simulink model "feedback_control"  (R2024a)
settings: Solver=FixedStepDiscrete  StartTime=0.0  StopTime=Inf  FixedStep=T_sample_control  RelTol=1e-3  EnableMultiTasking=on
undefined symbols (not defined in the file): Down, GPTRIP1SEL, T_sample_control, TZ1, Up
libraries: c2802xlib x7, c280xlib x4, c2837xDlib x4, simulink x3, mcbpositiondecoderlib x2, c2000lib x1
settings Model: DataDictionary=pid.sldd  EnableAccessToBaseWorkspace=off  ModifiedByFormat=The MathWorks Inc.  ExtModeTrigDuration=8  Creator=The MathWorks, Inc.  LastModifiedBy=The MathWorks Inc.
settings SolverCC: AlgebraicLoopSolver=TrustRegion  AutoInsertRateTranBlk=on
settings DataIOCC: SaveFormat=Array  ReturnWorkspaceOutputs=off
settings OptimizationCC: DefaultUnderspecifiedDataType=single  EnhancedBackFolding=on  PassReuseOutputArgsAs=Individual arguments  ExpressionDepthLimit=2147483647  EfficientFloat2IntCast=on  LifeSpan=1  MaxStackSize=1024  OptimizeBlockOrder=speed  DifferentSizesBufferReuse=on  OptimizationCustomize=off  EfficientTunableParamExpr=on
settings DebuggingCC: SolverPrmCheckMsg=warning  ParamSuppressDoubleToSinglePrecisionLossMsg=on  FcnCallInpInsideContextMsg=warning  UnconnectedInputMsg=warning  UnconnectedOutputMsg=warning  UnconnectedLineMsg=warning  UniqueDataStoreMsg=error  AssertControl=DisableAll  AllowSymbolicDim=off  StateNameClashWarn=warning  StrictBusMsg=ErrorOnBusTreatedAsVector  SFUnexpectedBacktrackingDiag=warning  SFNoUnconditionalDefaultTransitionDiag=warning  SFExecutionAtInitializationDiag=none  ArithmeticOperatorsInVariantConditions=warning
settings HardwareCC: ProdBitPerChar=16  ProdBitPerInt=16  ProdBitPerPointer=32  ProdBitPerSizeT=32  ProdBitPerPtrDiffT=32  ProdLargestAtomicInteger=Integer  ProdLargestAtomicFloat=None  ProdWordSize=16  ProdLongLongMode=on  ProdHWDeviceType=Texas Instruments->C2000  HardwareBoardFeatureSet=SoCBlockset
settings ModelReferenceCC: EnableRefExpFcnMdlSchedulingChecks=on  PropagateSignalLabelsOutOfModel=off
settings SFSimCC: SimUseLocalCustomCode=off  CustomCodeUndefinedFunction=UseInterfaceOnly
settings RTWCC: Description=Embedded Coder  SystemTargetFile=ert.tlc  HardwareBoard=TI Delfino F28379D LaunchPad  TemplateMakefile=ert_default_tmf  RTWUseLocalCustomCode=off  Toolchain=Texas Instruments Code Composer Studio (C2000)  IncludeHyperlinkInReport=on  CodeProfilingSaveOptions=MetricsOnly  GPUComputeCapability=3.5
settings CodeAppCC: IgnoreCustomStorageClasses=off  CustomSymbolStrType=$N$R$M  StateflowObjectComments=on  InternalIdentifier=Classic
settings ERTTargetCC: CodeReplacementLibrary=TI C28x  MultiwordLength=2048  ParenthesesLevel=Maximum  ExtModeTransport=4  ExtModeStaticAlloc=on  ExtModeAutomaticAllocSize=off  ExtModeStaticAllocSize=10000  ExtModeMexFile=ext_xcp  ExtModeIntrfLevel=Level2 - Open  ConvertIfToSwitch=off  SuppressUnreachableDefaultCases=off
settings ConfigComp: CovMetricSettings=dw  CovSaveCumulativeToWorkspaceVar=on  CovSaveSingleToWorkspaceVar=on  CovExternalEMLEnable=off  CovSFcnEnable=off

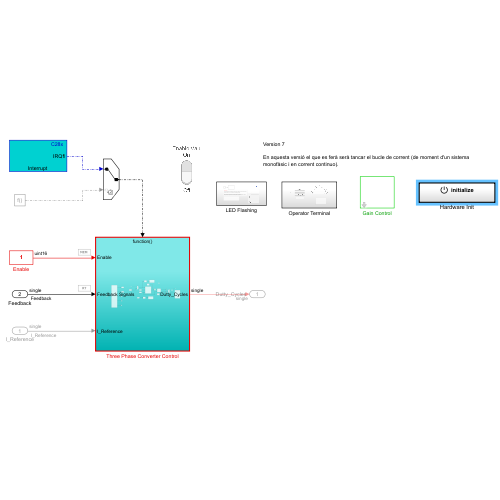
[thumbnail: Simulink's stored preview of the top-level diagram]
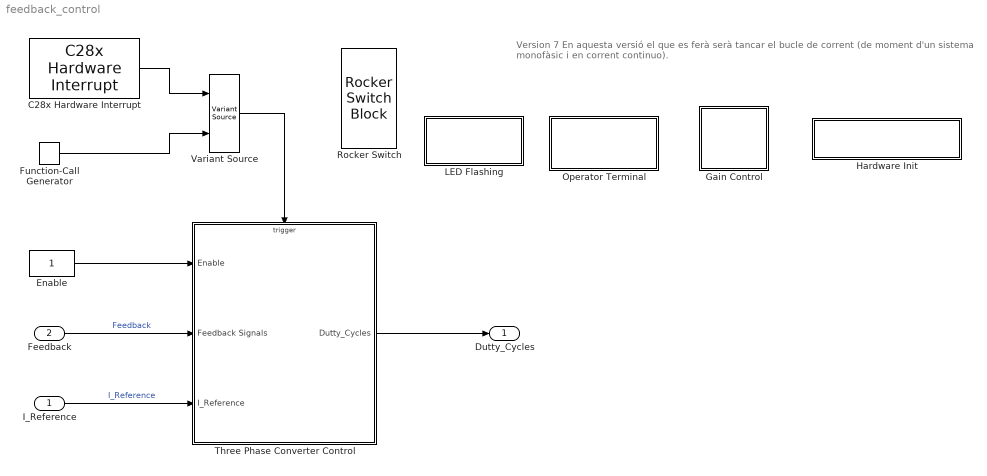
== system feedback_control ==
  note: Version 7
      |
      | En aquesta versió el que es ferà serà tancar el bucle de corrent (de moment d'un sistema monofàsic i en corrent continuo).
  I_Reference : Inport  OutDataTypeStr=single  PortDimensions=1  SampleTime=T_sample_control
  Feedback : Inport  Port=2  OutDataTypeStr=single  PortDimensions=3  SampleTime=T_sample_control
  C28x Hardware Interrupt : c2000lib/Scheduling/C28x Hardware Interrupt  irqnumbers=[1]  pienumbers=[1]  irqpriorities=[30]  irqpreempts=[1]  showinput=off  dspchiptype=C280X
  Enable : Constant  OutDataTypeStr=Inherit: Inherit via back propagation  SampleTime=-1
  Function-Call Generator : simulink/Ports & Subsystems/Function-Call Generator  sample_time=1/10000  numberOfIterations=1  DisallowWideOutput=off
  Gain Control : Subsystem  mask{Gain_Text_R=80 V/V, Gain_Text_S=80 V/V, Gain_Text_T=80 V/V}
      mask prompts: Gain_Text_R "Gain V/V:"; Gain_Text_S "Gain V/V:"; Gain_Text_T "Gain V/V:"
      mask init:
      | Gain_R = Gain_Text_R - 1;
      | Gain_S = Gain_Text_S - 1;
      | Gain_T = Gain_Text_T - 1;
      mask TypeOptions Gain_Text_R: 10 V/V | 20 V/V | 40 V/V | 80 V/V
      mask TypeOptions Gain_Text_S: 10 V/V | 20 V/V | 40 V/V | 80 V/V
      mask TypeOptions Gain_Text_T: 10 V/V | 20 V/V | 40 V/V | 80 V/V
  Hardware Init : Subsystem  TreatAsAtomicUnit=on
  LED Flashing : Subsystem
  Operator Terminal : Subsystem
  Rocker Switch : RockerSwitchBlock
      settings: Values={{'Off', 'On'}, [0 1]}
  Three Phase Converter Control : Subsystem
  Variant Source : VariantSource  VariantControlMode=sim codegen switching  OutputFunctionCall=on
  Dutty_Cycles : Outport  OutDataTypeStr=single  PortDimensions=3  SampleTime=T_sample_control
  wires:
  I_Reference/1 -> Three Phase Converter Control/3(I_Reference)  "I_Reference"
  Enable/1 -> Three Phase Converter Control/1(Enable)
  Feedback/1 -> Three Phase Converter Control/2(Feedback Signals)  "Feedback"
  Three Phase Converter Control/1(Dutty_Cycles) -> Dutty_Cycles/1
  C28x Hardware Interrupt/1 -> Variant Source/1
  Function-Call Generator/1 -> Variant Source/2
  Variant Source/1 -> Three Phase Converter Control/Trigger

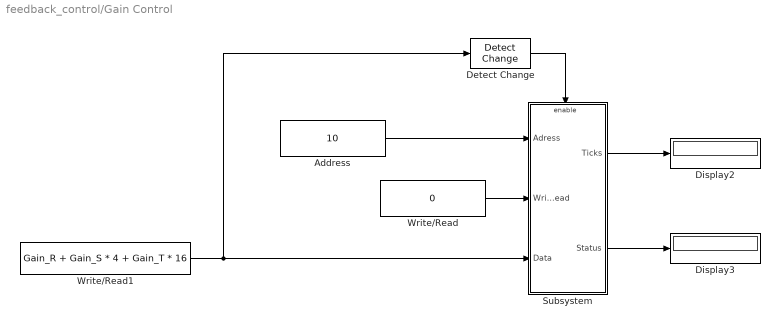
== system feedback_control/Gain Control ==
  Address : Constant  Value=10  OutDataTypeStr=uint16  SampleTime=-1
  Detect Change : simulink/Logic and Bit Operations/Detect Change  vinit=0  OutDataTypeStr=boolean
  Display2 : Display
  Display3 : Display
  Subsystem : Subsystem
  Write/Read : Constant  Value=0  OutDataTypeStr=uint16  SampleTime=-1
  Write/Read1 : Constant  Value=Gain_R + Gain_S * 4 + Gain_T * 16  OutDataTypeStr=uint16  SampleTime=-1
  wires:
  Detect Change/1 -> Subsystem/Enable
  Write/Read1/1 -> Detect Change/1, Subsystem/3(Data)
  Write/Read/1 -> Subsystem/2(Write/Read)
  Subsystem/2(Status) -> Display3/1
  Subsystem/1(Ticks) -> Display2/1
  Address/1 -> Subsystem/1(Adress)

== system feedback_control/Hardware Init ==
  Event Listener : EventListener  DisableCoverage=on  EventName=reset
  HW_Init : Subsystem  Variant=on  VariantControlMode=sim codegen switching

== system feedback_control/LED Flashing ==
  note: In the GPIO DO (Digital Output) instruction, a part from selecting the GPIO31, we will select the Toggle GPIO31, which means that every time we write a 1 to the position of the corresponding GPIO, it will toggle it state.
  note: Flashing LED
      |
      | The Launchpad used in this laboratory, has a blue LED, which we will turn on and off at a frequency of 2 Hz (every 1/2 second, the LED will trogle it state).
      |
      | At the figure at your right, there is the schematic of the Launchpad, where one can see that the LED D10 is connected to the GPIO31 ( General Purpose I/O ).
  Constant : Constant  OutDataTypeStr=single  SampleTime=0.5
  Digital Output1 : c2837xDlib/Digital Output  GPIO_Number=GPIO24~GPIO31  GPIO_Bit0=off  GPIO_BIT0_Toggle=off  GPIO_Bit1=off  GPIO_BIT1_Toggle=off  GPIO_Bit2=off  GPIO_BIT2_Toggle=off  GPIO_Bit3=off  GPIO_BIT3_Toggle=off  GPIO_Bit4=off  GPIO_BIT4_Toggle=off  GPIO_Bit5=off  GPIO_BIT5_Toggle=off  GPIO_Bit6=off  GPIO_BIT6_Toggle=off  GPIO_Bit7=on  GPIO_BIT7_Toggle=on
  wires:
  Constant/1 -> Digital Output1/1

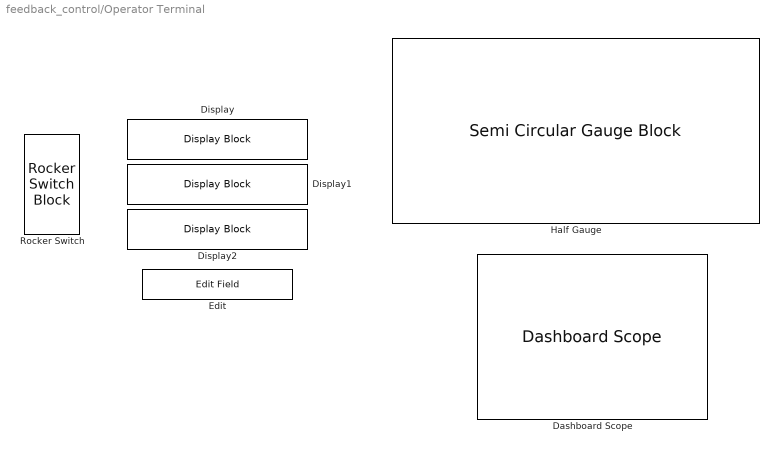
== system feedback_control/Operator Terminal ==
  Dashboard Scope : DashboardScope
  Display : DisplayBlock  Transparency=1
  Display1 : DisplayBlock  Transparency=1
  Display2 : DisplayBlock  Transparency=1
  Edit : EditField  LabelPosition=Hide  ShowInitialText=on  Alignment=Center
  Half Gauge : SemiCircularGaugeBlock  ScaleMax=50
  Rocker Switch : RockerSwitchBlock
      settings: Values={{'Off', 'On'}, [0 1]}

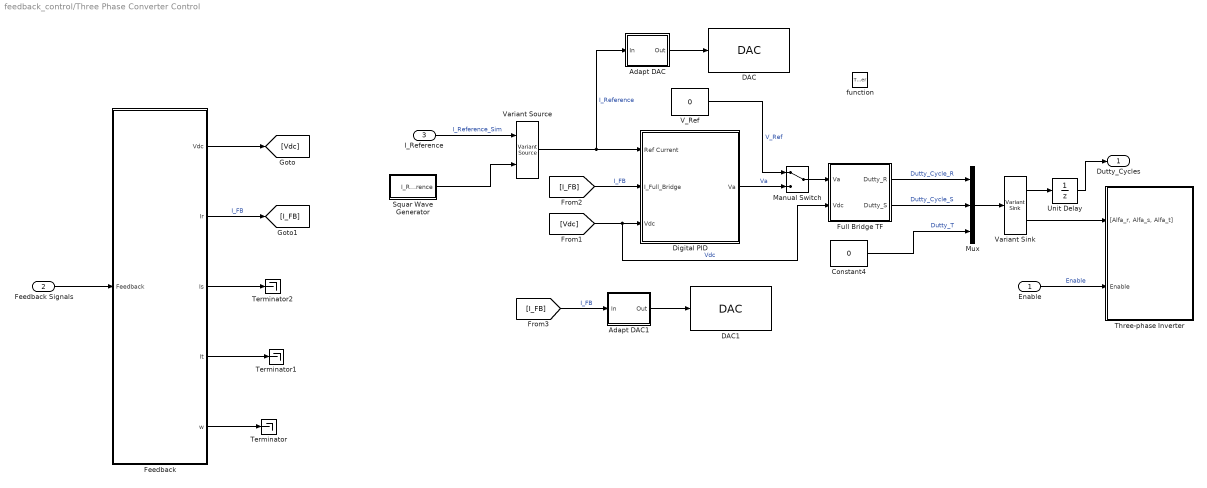
== system feedback_control/Three Phase Converter Control ==
  Enable : Inport
  Feedback Signals : Inport  Port=2
  I_Reference : Inport  Port=3
  function : TriggerPort  TriggerType=function-call  VariantControl=Variant  DisallowConstTsAndPrmTs=on
  Adapt DAC : Subsystem  mask{Offset=(3.3/3)*2048, Gain=(67.0/5.0)*(3/4095.0)}
  Adapt DAC1 : Subsystem  mask{Offset=2048, Gain=(2047*0.007*20*10)/1.65}
  Constant4 : Constant  Value=0  OutDataTypeStr=Inherit: Inherit via back propagation  SampleTime=-1
  DAC : c2837xDlib/DAC  channel=A  saturate=off
  DAC1 : c2837xDlib/DAC  channel=B  saturate=off
  Digital PID : Subsystem  mask{Kp=(2*15-1)*705e-3, Ki=2*15*15*705e-3*705e-3/9.05e-3, max=590, F=10}
      mask prompts: Kp "Proportional:"; Ki "Intragrator constant:"; max "Maximum Voltage:"; F "Sampling Frequency (hKz):"
      mask init:
      | Ts = 1 / (F * 1000);
  Feedback : Subsystem  Variant=on  VariantControlMode=sim codegen switching
  Full Bridge TF : Subsystem
  Manual Switch : ManualSwitch
  Mux : Mux  Inputs=3
  Squar Wave Generator : Subsystem
  Terminator : Terminator
  Terminator1 : Terminator
  Terminator2 : Terminator
  Three-phase Inverter : Subsystem  mask{Fcomm=10, FClk=100}
      mask prompts: Fcomm "Enter the Commutation Frequency (kHz):"; FClk "Enter the Clock Frequency of the CPU (MHz):"
      mask init:
      | Period = (FClk*1000)/(2*Fcomm);
  Unit Delay : UnitDelay  SampleTime=-1  HasFrameUpgradeWarning=on
  V_Ref : Constant  Value=0  OutDataTypeStr=Inherit: Inherit via back propagation  SampleTime=-1
  Variant Sink : VariantSink  VariantControlMode=sim codegen switching
  Variant Source : VariantSource  VariantControlMode=sim codegen switching
  Dutty_Cycles : Outport
  wires:
  [Vdc] -> Digital PID/3(Vdc), Full Bridge TF/2(Vdc)  "Vdc"
  Enable/1 -> Three-phase Inverter/2(Enable)  "Enable"
  Constant4/1 -> Mux/3  "Dutty_T"
  Variant Sink/2 -> Three-phase Inverter/1("[Alfa_r, Alfa_s, Alfa_t]")
  Feedback Signals/1 -> Feedback/1(Feedback)
  Variant Sink/1 -> Unit Delay/1
  Variant Source/1 -> Digital PID/1(Ref Current), Adapt DAC/1(In)  "I_Reference"
  Feedback/2(Ir) -> [I_FB]  "I_FB"
  Feedback/3(Is) -> Terminator2/1
  Feedback/4(It) -> Terminator1/1
  Feedback/5(w) -> Terminator/1
  Mux/1 -> Variant Sink/1
  Full Bridge TF/1(Dutty_R) -> Mux/1  "Dutty_Cycle_R"
  Full Bridge TF/2(Dutty_S) -> Mux/2  "Dutty_Cycle_S"
  Feedback/1(Vdc) -> [Vdc]
  [I_FB] -> Digital PID/2(I_Full_Bridge)  "I_FB"
  Unit Delay/1 -> Dutty_Cycles/1
  I_Reference/1 -> Variant Source/1  "I_Reference_Sim"
  Squar Wave Generator/1(I_Reference) -> Variant Source/2
  Digital PID/1(Va) -> Manual Switch/2  "Va"
  Manual Switch/1 -> Full Bridge TF/1(Va)
  V_Ref/1 -> Manual Switch/1  "V_Ref"
  Adapt DAC/1(Out) -> DAC/1
  Adapt DAC1/1(Out) -> DAC1/1
  [I_FB] -> Adapt DAC1/1(In)  "I_FB"

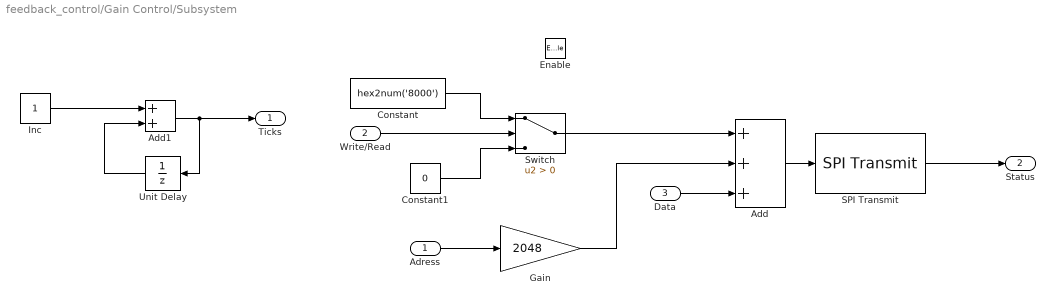
== system feedback_control/Gain Control/Subsystem ==
  Adress : Inport
  Write/Read : Inport  Port=2
  Data : Inport  Port=3
  Enable : EnablePort
  Add : Sum  Inputs=+++  AccumDataTypeStr=uint16
  Add1 : Sum
  Constant : Constant  Value=hex2num('8000')  OutDataTypeStr=uint16  SampleTime=-1
  Constant1 : Constant  Value=0  OutDataTypeStr=uint16  SampleTime=-1
  Gain : Gain  Gain=2048  ParamDataTypeStr=uint16  OutDataTypeStr=uint16
  Inc : Constant  OutDataTypeStr=uint16  SampleTime=-1
  SPI Transmit : c280xlib/SPI Transmit  SPISelect=SPI_A  ClockPolarity=Rising_edge  ClockPhase=No_delay  SPIModule=uint32(0)  Mode=Master  BusSpeed=uint32(1000000)  FirstBitToTransfer=Most significant bit (MSB)  ClockMode=0  BlockFunction=Write  EnableRegisterAddress=on  RegisterAddress=0  OutputDataType=int8  OutputDataLength=1  BlockingMode=off  DataBits=16  UseCustomSSPin=Provided by the SPI peripheral  ActiveLowSSPin=Active low  Pin=0
  Switch : Switch  Criteria=u2 > Threshold  SaturateOnIntegerOverflow=off  InputSameDT=off
  Unit Delay : UnitDelay  SampleTime=-1  StateName=Ticks  HasFrameUpgradeWarning=on
  Ticks : Outport  VectorParamsAs1DForOutWhenUnconnected=off
  Status : Outport  Port=2  VectorParamsAs1DForOutWhenUnconnected=off
  wires:
  Constant1/1 -> Switch/3
  Constant/1 -> Switch/1
  Write/Read/1 -> Switch/2
  Adress/1 -> Gain/1
  Switch/1 -> Add/1
  Gain/1 -> Add/2
  Add/1 -> SPI Transmit/1
  SPI Transmit/1 -> Status/1
  Add1/1 -> Ticks/1, Unit Delay/1
  Unit Delay/1 -> Add1/2
  Inc/1 -> Add1/1
  Data/1 -> Add/3

== system feedback_control/Hardware Init/HW_Init ==
  HW_Init (Codegen) : Subsystem  VariantControl=(codegen)
  HW_Init (sim) : Subsystem  VariantControl=(sim)

== system feedback_control/Three Phase Converter Control/Adapt DAC ==
  In : Inport
  Add : Sum
  Data Type Conversion : DataTypeConversion  SaturateOnIntegerOverflow=off  RndMeth=Floor
  Gain2 : Gain  Gain=Gain  OutDataTypeStr=single
  Offset : Constant  Value=Offset  OutDataTypeStr=single  SampleTime=-1
  Out : Outport
  wires:
  Offset/1 -> Add/2
  In/1 -> Data Type Conversion/1
  Add/1 -> Out/1
  Gain2/1 -> Add/1
  Data Type Conversion/1 -> Gain2/1

== system feedback_control/Three Phase Converter Control/Adapt DAC1 ==
  In : Inport
  Add : Sum  Inputs=+-
  Data Type Conversion : DataTypeConversion  SaturateOnIntegerOverflow=off  RndMeth=Floor
  Gain2 : Gain  Gain=Gain  OutDataTypeStr=single
  Offset : Constant  Value=Offset  OutDataTypeStr=single  SampleTime=-1
  Out : Outport
  wires:
  Data Type Conversion/1 -> Gain2/1
  Gain2/1 -> Add/1
  Add/1 -> Out/1
  In/1 -> Data Type Conversion/1
  Offset/1 -> Add/2

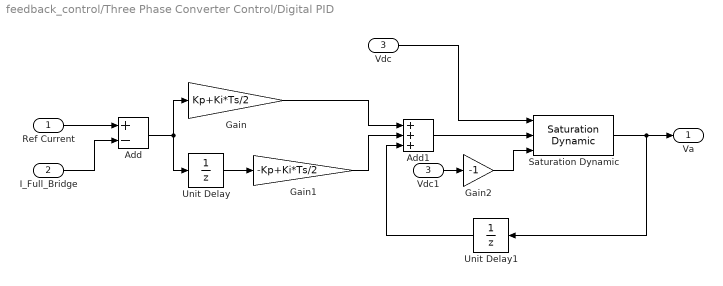
== system feedback_control/Three Phase Converter Control/Digital PID ==
  Ref Current : Inport
  I_Full_Bridge : Inport  Port=2
  Vdc : Inport  Port=3
  Add : Sum  Inputs=+-
  Add1 : Sum  Inputs=+++
  Gain : Gain  Gain=Kp+Ki*Ts/2
  Gain1 : Gain  Gain=-Kp+Ki*Ts/2
  Gain2 : Gain  Gain=-1
  Saturation Dynamic : simulink/Discontinuities/Saturation Dynamic  OutMin=[]  OutMax=[]  OutDataTypeStr=Inherit: Inherit via back propagation  OutDataType=fixdt(1, 16)  OutScaling=2^-10  DoSatur=off
  Unit Delay : UnitDelay  SampleTime=-1  HasFrameUpgradeWarning=on
  Unit Delay1 : UnitDelay  SampleTime=-1  HasFrameUpgradeWarning=on
  Vdc1 : InportShadow  Port=3
  Va : Outport  PortDimensions=1
  wires:
  Unit Delay/1 -> Gain1/1
  Add/1 -> Gain/1, Unit Delay/1
  Gain/1 -> Add1/1
  Gain1/1 -> Add1/2
  Add1/1 -> Saturation Dynamic/2
  Saturation Dynamic/1 -> Unit Delay1/1, Va/1
  Ref Current/1 -> Add/1
  I_Full_Bridge/1 -> Add/2
  Unit Delay1/1 -> Add1/3
  Vdc/1 -> Saturation Dynamic/1
  Vdc1/1 -> Gain2/1
  Gain2/1 -> Saturation Dynamic/3

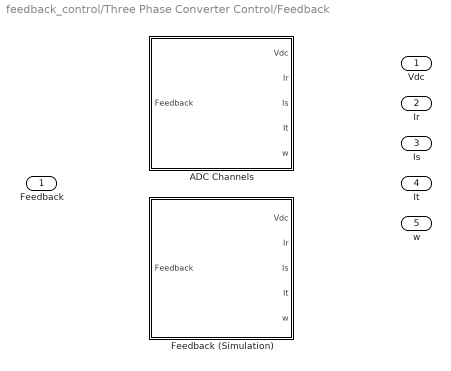
== system feedback_control/Three Phase Converter Control/Feedback ==
  Feedback : Inport
  ADC Channels : Subsystem  VariantControl=(codegen)
  Feedback (Simulation) : Subsystem  VariantControl=(sim)
  Vdc : Outport
  Ir : Outport  Port=2
  Is : Outport  Port=3
  It : Outport  Port=4
  w : Outport  Port=5

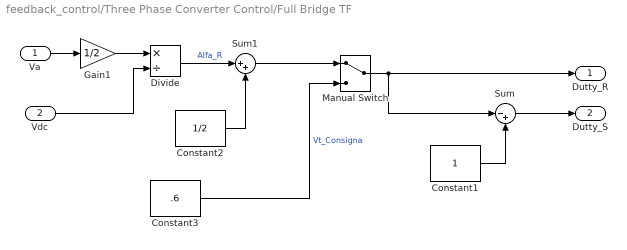
== system feedback_control/Three Phase Converter Control/Full Bridge TF ==
  Va : Inport
  Vdc : Inport  Port=2
  Constant1 : Constant  OutDataTypeStr=Inherit: Inherit via back propagation  SampleTime=-1
  Constant2 : Constant  Value=1/2  OutDataTypeStr=Inherit: Inherit via back propagation  SampleTime=-1
  Constant3 : Constant  Value=.6  OutDataTypeStr=Inherit: Inherit via back propagation  SampleTime=-1
  Divide : Product  Inputs=*/
  Gain1 : Gain  Gain=1/2  OutDataTypeStr=Inherit: Same as input
  Manual Switch : ManualSwitch
  Sum : Sum  Inputs=|-+
  Sum1 : Sum  Inputs=|++
  Dutty_R : Outport
  Dutty_S : Outport  Port=2
  wires:
  Va/1 -> Gain1/1
  Sum/1 -> Dutty_S/1
  Constant3/1 -> Manual Switch/2  "Vt_Consigna"
  Sum1/1 -> Manual Switch/1
  Constant1/1 -> Sum/2
  Manual Switch/1 -> Sum/1, Dutty_R/1
  Gain1/1 -> Divide/1
  Vdc/1 -> Divide/2
  Divide/1 -> Sum1/1  "Alfa_R"
  Constant2/1 -> Sum1/2

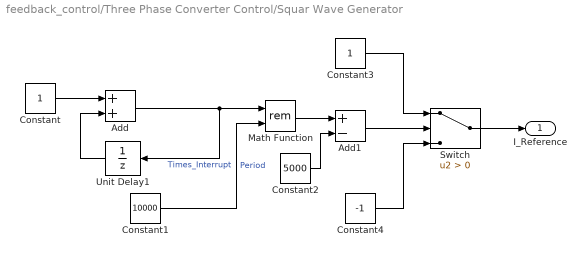
== system feedback_control/Three Phase Converter Control/Squar Wave Generator ==
  Add : Sum
  Add1 : Sum  Inputs=+-
  Constant : Constant  OutDataTypeStr=uint32
  Constant1 : Constant  Value=10000  OutDataTypeStr=uint32
  Constant2 : Constant  Value=5000  OutDataTypeStr=uint32
  Constant3 : Constant  OutDataTypeStr=Inherit: Inherit via back propagation
  Constant4 : Constant  Value=-1  OutDataTypeStr=Inherit: Inherit via back propagation
  Math Function : Math  Operator=rem
  Switch : Switch  Criteria=u2 > Threshold  SaturateOnIntegerOverflow=off  InputSameDT=off
  Unit Delay1 : UnitDelay  SampleTime=-1  HasFrameUpgradeWarning=on
  I_Reference : Outport
  wires:
  Constant1/1 -> Math Function/2  "Period"
  Constant/1 -> Add/1
  Add/1 -> Math Function/1, Unit Delay1/1  "Times_Interrupt"
  Unit Delay1/1 -> Add/2
  Math Function/1 -> Add1/1
  Constant2/1 -> Add1/2
  Add1/1 -> Switch/2
  Switch/1 -> I_Reference/1
  Constant4/1 -> Switch/3
  Constant3/1 -> Switch/1

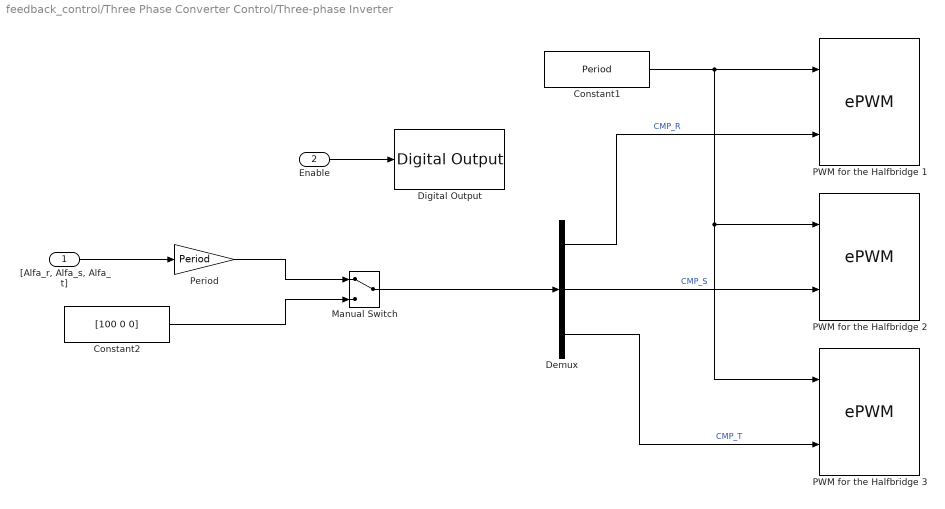
== system feedback_control/Three Phase Converter Control/Three-phase Inverter ==
  "[Alfa_r, Alfa_s, Alfa_t]" : Inport
  Enable : Inport  Port=2  OutDataTypeStr=uint16
  Constant1 : Constant  Value=Period  OutDataTypeStr=single  SampleTime=-1
  Constant2 : Constant  Value=[100 0 0]  OutDataTypeStr=Inherit: Inherit via back propagation  SampleTime=-1
  Demux : Demux  Outputs=3
  Digital Output : c2837xDlib/Digital Output  GPIO_Number=GPIO120~GPIO127  GPIO_Bit0=off  GPIO_BIT0_Toggle=off  GPIO_Bit1=off  GPIO_BIT1_Toggle=off  GPIO_Bit2=off  GPIO_BIT2_Toggle=off  GPIO_Bit3=off  GPIO_BIT3_Toggle=off  GPIO_Bit4=on  GPIO_BIT4_Toggle=off  GPIO_Bit5=off  GPIO_BIT5_Toggle=off  GPIO_Bit6=off  GPIO_BIT6_Toggle=off  GPIO_Bit7=off  GPIO_BIT7_Toggle=off
  Manual Switch : ManualSwitch
  PWM for the Halfbridge 1 : c2802xlib/ePWM  PwmType=C2000_Type4  useModule=ePWM1  ePWMxLINKTBPRD=Not Linked  periodUnits=Clock cycles  timerSource=Input port  timerPeriod_clk=Period/2  timerPeriod_sec=0.0001  tbshadow=Counter equals to zero  countingMode=Up-Down  phaseActiveEnable=Disable  phaseDirection=Count down after sync  phaseActive=0  synchronizationEnable=off  dcaevt1Sync=off  dcbevt1Sync=off  synchronizationOption=Counter equals to zero (CTR=Zero)  dcbevt1SyncOut=off  dcaevt1SyncOut=off  cmpdSyncOut=off  cmpcSyncOut=off  cmpbSyncOut=off  zeroSyncOut=off  swfSyncOut=off  perSynchronizationOption=Counter equals to period (CTR=PRD)  clockPrescale=1  HSclockPrescale=1  enswap=off  ePWMxAStatus=on  ePWMxAactionLogic1=Set  ePWMxAactionLogic2=Clear  ePWMxAactionLogic3=Clear  ePWMxAactionLogic4=Set  ePWMxAactionLogic5=Do nothing  ePWMxAactionLogic6=Do nothing  ePWMxACSFenable=off  ePWMxACSFvalue=Forcing disable  ePWMxASFreload=Zero  ePWMxBStatus=off  ePWMxBactionLogic1=Set  ePWMxBactionLogic2=Clear  ePWMxBactionLogic3=Do nothing  ePWMxBactionLogic4=Do nothing  ePWMxBactionLogic5=Clear  ePWMxBactionLogic6=Set  ePWMxBCSFenable=off  ePWMxBCSFvalue=Forcing disable  ePWMxBSFreload=Zero  ePWNxBOutWay=off  ePWMxLINKCMPA=Not Linked  CMPAUnits=Clock cycles  CMPASource=Input port  CMPAValue_per=50  CMPAValue_clk=Period/2  enCMPAshadow=Counter equals to zero or period (CTR=Zero or CTR=PRD)  ePWMxLINKCMPB=Not Linked  CMPBUnits=Clock cycles  CMPBSource=Specify via dialog  CMPBValue_per=50  CMPBValue_clk=32000  enCMPBshadow=Counter equals to zero (CTR=Zero)  ePWMxLINKCMPC=Not Linked  CMPCUnits=Clock cycles  CMPCSource=Specify via dialog  CMPCValue_per=50  CMPCValue_clk=32000  enCMPCshadow=Counter equals to zero (CTR=Zero)  ePWMxLINKCMPD=Not Linked  CMPDUnits=Clock cycles  CMPDSource=Specify via dialog  CMPDValue_per=50  CMPDValue_clk=32000  enCMPDshadow=Counter equals to zero (CTR=Zero)  enableDBePWMxA=on  enableDBePWMxB=on  enhalfcycle=off  DBpolarity=Active high complementary (AHC)  DBedgeDelay=Positive  DBSource_ePWMxA=ePWMxA  DBSource_ePWMxB=ePWMxA  DBPeriodUnits=Clock cycles  DBperiodSource=Specify via dialog  REDperiod=20  FEDperiod=20  REDperiod_sec=0  FEDperiod_sec=0  LoadModeDBRED=Immediate without using shadow  LoadModeDBFED=Immediate without using shadow  adcstartModuleA=on  adcrequestEventA=First event  adcstartEventA=Digital Compare Module A Event 1 start of conversion (DCAEVT1.soc)  adcstartEventA_type2=Counter equals to period (CTR=PRD)  adcstartModuleB=off  adcrequestEventB=First event  adcstartEventB=Counter equals to zero (CTR=Zero)  adcstartEventB_type2=Counter equals to zero (CTR=Zero)  intEn=off  intPrd=First event  intSel=Counter equals to zero (CTR=Zero)  intSel_type2=Counter equals to zero (CTR=Zero)  hrpe=off  enHRPWM=off  HRPWM_LoadMode=Counter equals to period (CTR=PRD)  HRPWM_CTLMode=Duty or Period control mode  HRPWM_EDGMode=Both edge  hrpeb=off  enHRPWMB=off  HRPWM_LoadModeB=Counter equals to zero (CTR=ZERO)  HRPWM_CTLModeB=Duty or Period control mode  HRPWM_EDGModeB=Both edge  enHRDBRED=off  enHRDBFED=off  enSFO=on  enautoconv=on  chopperEnable=off  chopperFrequency=1  chopperFirstwidth=1  chopperDuty=12.5%  tripZonesource=Specify via dialog  tzselOSHT1=off  tzselOSHT2=off  tzselOSHT3=off  tzselOSHT4=off  tzselOSHT5=off  tzselOSHT6=off  tzselOSHDCAEV1=off  tzselOSHDCBEV1=off  tzselCBC1=off  tzselCBC2=off  tzselCBC3=off  tzselCBC4=off  tzselCBC5=off  tzselCBC6=off  tzselCBCDCAEV2=off  tzselCBCDCBEV2=off  enTzOstIntr=off  enTzCbcIntr=off  enTzDCAEVT1Intr=off  enTzDCAEVT2Intr=off  enTzDCBEVT1Intr=off  enTzDCBEVT2Intr=off  tzclrCBCLatch=Counter equals to zero (CTR=Zero)  ePWMxAforced=No action  ePWMxBforced=No action  DCAEVT1forced=No action  DCBEVT1forced=No action  DCAEVT2forced=No action  DCBEVT2forced=No action  dcah=Trip Zone 1 input (TZ1)  dcal=Trip Zone 2 input (TZ2)  dcbh=Trip Zone 1 input (TZ1)  dcbl=Trip Zone 2 input (TZ2)  dcah_type2=GPTRIP1SEL/(TZ1)  dcal_type2=GPTRIP1SEL/(TZ1)  dcbh_type2=GPTRIP1SEL/(TZ1)  dcbl_type2=GPTRIP1SEL/(TZ1)  gendcaevt1=Event disabled  gendcaevt2=Event disabled  gendcbevt1=Event disabled  gendcbevt2=Event disabled  dcaevt1src=DCAEVT1 with sync  dcaevt2src=DCAEVT2 with sync  dcbevt1src=DCBEVT1 with sync  dcbevt2src=DCBEVT2 with sync  pulsesel=Counter equals to zero (CTR=Zero)  blankinv=off  blankoffset=0  blankwidth=0  evsrcsel=Filtered version of DCAEVT1 (DCAEVT1FILT)  encape=off
      settings: LibrarySourceBlock=c2837xDlib/ePWM
  PWM for the Halfbridge 2 : c2802xlib/ePWM  PwmType=C2000_Type4  useModule=ePWM2  ePWMxLINKTBPRD=Not Linked  periodUnits=Clock cycles  timerSource=Input port  timerPeriod_clk=Period/2  timerPeriod_sec=0.0001  tbshadow=Counter equals to zero  countingMode=Up-Down  phaseActiveEnable=Set counter to phase value specified via dialog  phaseDirection=Count up after sync  phaseActive=0  synchronizationEnable=off  dcaevt1Sync=off  dcbevt1Sync=off  synchronizationOption=Pass through (EPWMxSYNCI or SWFSYNC)  dcbevt1SyncOut=off  dcaevt1SyncOut=off  cmpdSyncOut=off  cmpcSyncOut=off  cmpbSyncOut=off  zeroSyncOut=off  swfSyncOut=off  perSynchronizationOption=Counter equals to period (CTR=PRD)  clockPrescale=1  HSclockPrescale=1  enswap=off  ePWMxAStatus=on  ePWMxAactionLogic1=Set  ePWMxAactionLogic2=Clear  ePWMxAactionLogic3=Clear  ePWMxAactionLogic4=Set  ePWMxAactionLogic5=Do nothing  ePWMxAactionLogic6=Do nothing  ePWMxACSFenable=off  ePWMxACSFvalue=Forcing disable  ePWMxASFreload=Zero  ePWMxBStatus=off  ePWMxBactionLogic1=Set  ePWMxBactionLogic2=Clear  ePWMxBactionLogic3=Do nothing  ePWMxBactionLogic4=Do nothing  ePWMxBactionLogic5=Clear  ePWMxBactionLogic6=Set  ePWMxBCSFenable=off  ePWMxBCSFvalue=Forcing disable  ePWMxBSFreload=Zero  ePWNxBOutWay=off  ePWMxLINKCMPA=Not Linked  CMPAUnits=Clock cycles  CMPASource=Input port  CMPAValue_per=50  CMPAValue_clk=Period/2  enCMPAshadow=Counter equals to zero or period (CTR=Zero or CTR=PRD)  ePWMxLINKCMPB=Not Linked  CMPBUnits=Clock cycles  CMPBSource=Specify via dialog  CMPBValue_per=50  CMPBValue_clk=32000  enCMPBshadow=Counter equals to zero (CTR=Zero)  ePWMxLINKCMPC=Not Linked  CMPCUnits=Clock cycles  CMPCSource=Specify via dialog  CMPCValue_per=50  CMPCValue_clk=32000  enCMPCshadow=Counter equals to zero (CTR=Zero)  ePWMxLINKCMPD=Not Linked  CMPDUnits=Clock cycles  CMPDSource=Specify via dialog  CMPDValue_per=50  CMPDValue_clk=32000  enCMPDshadow=Counter equals to zero (CTR=Zero)  enableDBePWMxA=on  enableDBePWMxB=on  enhalfcycle=off  DBpolarity=Active high complementary (AHC)  DBedgeDelay=Positive  DBSource_ePWMxA=ePWMxA  DBSource_ePWMxB=ePWMxA  DBPeriodUnits=Clock cycles  DBperiodSource=Specify via dialog  REDperiod=20  FEDperiod=20  REDperiod_sec=0  FEDperiod_sec=0  LoadModeDBRED=Immediate without using shadow  LoadModeDBFED=Immediate without using shadow  adcstartModuleA=off  adcrequestEventA=First event  adcstartEventA=Digital Compare Module A Event 1 start of conversion (DCAEVT1.soc)  adcstartEventA_type2=Counter equals to zero (CTR=Zero)  adcstartModuleB=off  adcrequestEventB=First event  adcstartEventB=Counter equals to zero (CTR=Zero)  adcstartEventB_type2=Counter equals to zero (CTR=Zero)  intEn=off  intPrd=First event  intSel=Counter equals to zero (CTR=Zero)  intSel_type2=Counter equals to zero (CTR=Zero)  hrpe=off  enHRPWM=off  HRPWM_LoadMode=Counter equals to period (CTR=PRD)  HRPWM_CTLMode=Duty or Period control mode  HRPWM_EDGMode=Both edge  hrpeb=off  enHRPWMB=off  HRPWM_LoadModeB=Counter equals to zero (CTR=ZERO)  HRPWM_CTLModeB=Duty or Period control mode  HRPWM_EDGModeB=Both edge  enHRDBRED=off  enHRDBFED=off  enSFO=on  enautoconv=on  chopperEnable=off  chopperFrequency=1  chopperFirstwidth=1  chopperDuty=12.5%  tripZonesource=Specify via dialog  tzselOSHT1=off  tzselOSHT2=off  tzselOSHT3=off  tzselOSHT4=off  tzselOSHT5=off  tzselOSHT6=off  tzselOSHDCAEV1=off  tzselOSHDCBEV1=off  tzselCBC1=off  tzselCBC2=off  tzselCBC3=off  tzselCBC4=off  tzselCBC5=off  tzselCBC6=off  tzselCBCDCAEV2=off  tzselCBCDCBEV2=off  enTzOstIntr=off  enTzCbcIntr=off  enTzDCAEVT1Intr=off  enTzDCAEVT2Intr=off  enTzDCBEVT1Intr=off  enTzDCBEVT2Intr=off  tzclrCBCLatch=Counter equals to zero (CTR=Zero)  ePWMxAforced=No action  ePWMxBforced=No action  DCAEVT1forced=No action  DCBEVT1forced=No action  DCAEVT2forced=No action  DCBEVT2forced=No action  dcah=Trip Zone 1 input (TZ1)  dcal=Trip Zone 2 input (TZ2)  dcbh=Trip Zone 1 input (TZ1)  dcbl=Trip Zone 2 input (TZ2)  dcah_type2=GPTRIP1SEL/(TZ1)  dcal_type2=GPTRIP1SEL/(TZ1)  dcbh_type2=GPTRIP1SEL/(TZ1)  dcbl_type2=GPTRIP1SEL/(TZ1)  gendcaevt1=Event disabled  gendcaevt2=Event disabled  gendcbevt1=Event disabled  gendcbevt2=Event disabled  dcaevt1src=DCAEVT1 with sync  dcaevt2src=DCAEVT2 with sync  dcbevt1src=DCBEVT1 with sync  dcbevt2src=DCBEVT2 with sync  pulsesel=Counter equals to zero (CTR=Zero)  blankinv=off  blankoffset=0  blankwidth=0  evsrcsel=Filtered version of DCAEVT1 (DCAEVT1FILT)  encape=off
      settings: LibrarySourceBlock=c2837xDlib/ePWM
  PWM for the Halfbridge 3 : c2802xlib/ePWM  PwmType=C2000_Type4  useModule=ePWM3  ePWMxLINKTBPRD=Not Linked  periodUnits=Clock cycles  timerSource=Input port  timerPeriod_clk=Period/2  timerPeriod_sec=0.0001  tbshadow=Counter equals to zero  countingMode=Up-Down  phaseActiveEnable=Set counter to phase value specified via dialog  phaseDirection=Count up after sync  phaseActive=0  synchronizationEnable=off  dcaevt1Sync=off  dcbevt1Sync=off  synchronizationOption=Pass through (EPWMxSYNCI or SWFSYNC)  dcbevt1SyncOut=off  dcaevt1SyncOut=off  cmpdSyncOut=off  cmpcSyncOut=off  cmpbSyncOut=off  zeroSyncOut=off  swfSyncOut=off  perSynchronizationOption=Counter equals to period (CTR=PRD)  clockPrescale=1  HSclockPrescale=1  enswap=off  ePWMxAStatus=on  ePWMxAactionLogic1=Set  ePWMxAactionLogic2=Clear  ePWMxAactionLogic3=Clear  ePWMxAactionLogic4=Set  ePWMxAactionLogic5=Do nothing  ePWMxAactionLogic6=Do nothing  ePWMxACSFenable=off  ePWMxACSFvalue=Forcing disable  ePWMxASFreload=Zero  ePWMxBStatus=off  ePWMxBactionLogic1=Set  ePWMxBactionLogic2=Clear  ePWMxBactionLogic3=Do nothing  ePWMxBactionLogic4=Do nothing  ePWMxBactionLogic5=Clear  ePWMxBactionLogic6=Set  ePWMxBCSFenable=off  ePWMxBCSFvalue=Forcing disable  ePWMxBSFreload=Zero  ePWNxBOutWay=off  ePWMxLINKCMPA=Not Linked  CMPAUnits=Clock cycles  CMPASource=Input port  CMPAValue_per=50  CMPAValue_clk=Period/2  enCMPAshadow=Counter equals to zero or period (CTR=Zero or CTR=PRD)  ePWMxLINKCMPB=Not Linked  CMPBUnits=Clock cycles  CMPBSource=Specify via dialog  CMPBValue_per=50  CMPBValue_clk=32000  enCMPBshadow=Counter equals to zero (CTR=Zero)  ePWMxLINKCMPC=Not Linked  CMPCUnits=Clock cycles  CMPCSource=Specify via dialog  CMPCValue_per=50  CMPCValue_clk=32000  enCMPCshadow=Counter equals to zero (CTR=Zero)  ePWMxLINKCMPD=Not Linked  CMPDUnits=Clock cycles  CMPDSource=Specify via dialog  CMPDValue_per=50  CMPDValue_clk=32000  enCMPDshadow=Counter equals to zero (CTR=Zero)  enableDBePWMxA=on  enableDBePWMxB=on  enhalfcycle=off  DBpolarity=Active high complementary (AHC)  DBedgeDelay=Positive  DBSource_ePWMxA=ePWMxA  DBSource_ePWMxB=ePWMxA  DBPeriodUnits=Clock cycles  DBperiodSource=Specify via dialog  REDperiod=20  FEDperiod=20  REDperiod_sec=0  FEDperiod_sec=0  LoadModeDBRED=Immediate without using shadow  LoadModeDBFED=Immediate without using shadow  adcstartModuleA=off  adcrequestEventA=First event  adcstartEventA=Digital Compare Module A Event 1 start of conversion (DCAEVT1.soc)  adcstartEventA_type2=Counter equals to zero (CTR=Zero)  adcstartModuleB=off  adcrequestEventB=First event  adcstartEventB=Counter equals to zero (CTR=Zero)  adcstartEventB_type2=Counter equals to zero (CTR=Zero)  intEn=off  intPrd=First event  intSel=Counter equals to zero (CTR=Zero)  intSel_type2=Counter equals to zero (CTR=Zero)  hrpe=off  enHRPWM=off  HRPWM_LoadMode=Counter equals to period (CTR=PRD)  HRPWM_CTLMode=Duty or Period control mode  HRPWM_EDGMode=Both edge  hrpeb=off  enHRPWMB=off  HRPWM_LoadModeB=Counter equals to zero (CTR=ZERO)  HRPWM_CTLModeB=Duty or Period control mode  HRPWM_EDGModeB=Both edge  enHRDBRED=off  enHRDBFED=off  enSFO=on  enautoconv=on  chopperEnable=off  chopperFrequency=1  chopperFirstwidth=1  chopperDuty=12.5%  tripZonesource=Specify via dialog  tzselOSHT1=off  tzselOSHT2=off  tzselOSHT3=off  tzselOSHT4=off  tzselOSHT5=off  tzselOSHT6=off  tzselOSHDCAEV1=off  tzselOSHDCBEV1=off  tzselCBC1=off  tzselCBC2=off  tzselCBC3=off  tzselCBC4=off  tzselCBC5=off  tzselCBC6=off  tzselCBCDCAEV2=off  tzselCBCDCBEV2=off  enTzOstIntr=off  enTzCbcIntr=off  enTzDCAEVT1Intr=off  enTzDCAEVT2Intr=off  enTzDCBEVT1Intr=off  enTzDCBEVT2Intr=off  tzclrCBCLatch=Counter equals to zero (CTR=Zero)  ePWMxAforced=No action  ePWMxBforced=No action  DCAEVT1forced=No action  DCBEVT1forced=No action  DCAEVT2forced=No action  DCBEVT2forced=No action  dcah=Trip Zone 1 input (TZ1)  dcal=Trip Zone 2 input (TZ2)  dcbh=Trip Zone 1 input (TZ1)  dcbl=Trip Zone 2 input (TZ2)  dcah_type2=GPTRIP1SEL/(TZ1)  dcal_type2=GPTRIP1SEL/(TZ1)  dcbh_type2=GPTRIP1SEL/(TZ1)  dcbl_type2=GPTRIP1SEL/(TZ1)  gendcaevt1=Event disabled  gendcaevt2=Event disabled  gendcbevt1=Event disabled  gendcbevt2=Event disabled  dcaevt1src=DCAEVT1 with sync  dcaevt2src=DCAEVT2 with sync  dcbevt1src=DCBEVT1 with sync  dcbevt2src=DCBEVT2 with sync  pulsesel=Counter equals to zero (CTR=Zero)  blankinv=off  blankoffset=0  blankwidth=0  evsrcsel=Filtered version of DCAEVT1 (DCAEVT1FILT)  encape=off
      settings: LibrarySourceBlock=c2837xDlib/ePWM
  Period : Gain  Gain=Period  ParamDataTypeStr=single
  wires:
  Demux/1 -> PWM for the Halfbridge 1/2  "CMP_R"
  Constant1/1 -> PWM for the Halfbridge 3/1, PWM for the Halfbridge 2/1, PWM for the Halfbridge 1/1
  Demux/2 -> PWM for the Halfbridge 2/2  "CMP_S"
  Demux/3 -> PWM for the Halfbridge 3/2  "CMP_T"
  Enable/1 -> Digital Output/1
  "[Alfa_r, Alfa_s, Alfa_t]"/1 -> Period/1
  Manual Switch/1 -> Demux/1
  Period/1 -> Manual Switch/1
  Constant2/1 -> Manual Switch/2

== system feedback_control/Hardware Init/HW_Init/HW_Init (Codegen) ==
  note: System Outputs
  note: Block priorities are set to ensure the sequence of operation.
  note: for BoostXL-DRV8305 connected to LaunchXL-28379D
  Enable DRV8305 for motor 1 : Subsystem  Priority=10  TreatAsAtomicUnit=on

== system feedback_control/Hardware Init/HW_Init/HW_Init (sim) ==

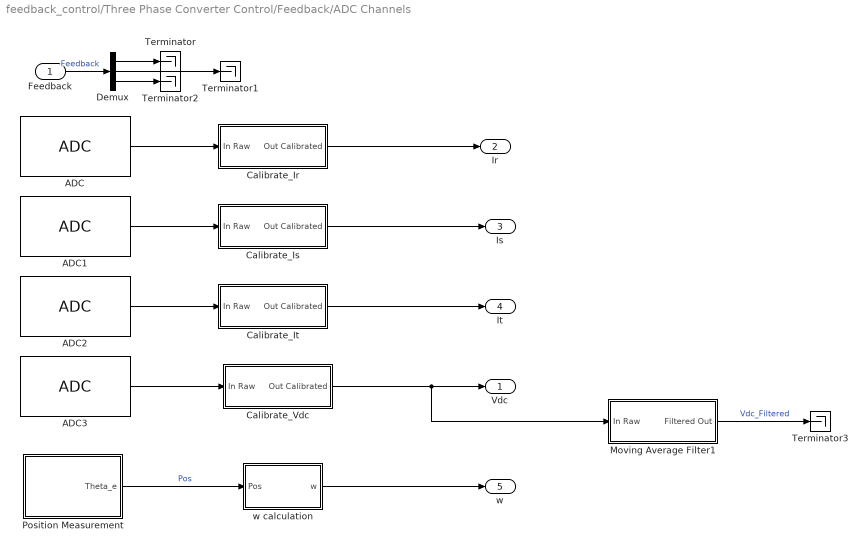
== system feedback_control/Three Phase Converter Control/Feedback/ADC Channels ==
  Feedback : Inport
  ADC : c2802xlib/ADC  blkParamProc=C2000_Type4  ADCModule=C  samplingMode=Single sample mode  ADCResolution=12-bit (Single-ended input)  useSOC1=SOC0  useSOC2=SOC0_SOC1  SOCAcquisitionWindow=15  SOCTriggerSource=ePWM1_ADCSOCA  SOCInterruptTrigger=No ADCINT  Ts=-1  dType=uint16  postInterrupt=off  interruptSel=ADCINT1  ADCINTContinuous=on  endma=off  chdma=1  conv1=ADCINA0  conv2=ADCINA0 and ADCINB0  conv1_Type4=ADCIN2  conv2_Type4=ADCIN0 and ADCIN1
      settings: LibrarySourceBlock=c2837xDlib/ADC
  ADC1 : c2802xlib/ADC  blkParamProc=C2000_Type4  ADCModule=B  samplingMode=Single sample mode  ADCResolution=12-bit (Single-ended input)  useSOC1=SOC1  useSOC2=SOC0_SOC1  SOCAcquisitionWindow=15  SOCTriggerSource=ePWM1_ADCSOCA  SOCInterruptTrigger=No ADCINT  Ts=-1  dType=uint16  postInterrupt=off  interruptSel=ADCINT1  ADCINTContinuous=on  endma=off  chdma=1  conv1=ADCINA0  conv2=ADCINA0 and ADCINB0  conv1_Type4=ADCIN2  conv2_Type4=ADCIN0 and ADCIN1
      settings: LibrarySourceBlock=c2837xDlib/ADC
  ADC2 : c2802xlib/ADC  blkParamProc=C2000_Type4  ADCModule=A  samplingMode=Single sample mode  ADCResolution=12-bit (Single-ended input)  useSOC1=SOC2  useSOC2=SOC0_SOC1  SOCAcquisitionWindow=15  SOCTriggerSource=ePWM1_ADCSOCA  SOCInterruptTrigger=No ADCINT  Ts=-1  dType=uint16  postInterrupt=off  interruptSel=ADCINT1  ADCINTContinuous=on  endma=off  chdma=1  conv1=ADCINA0  conv2=ADCINA0 and ADCINB0  conv1_Type4=ADCIN2  conv2_Type4=ADCIN0 and ADCIN1
      settings: LibrarySourceBlock=c2837xDlib/ADC
  ADC3 : c2802xlib/ADC  blkParamProc=C2000_Type4  ADCModule=A  samplingMode=Single sample mode  ADCResolution=12-bit (Single-ended input)  useSOC1=SOC3  useSOC2=SOC0_SOC1  SOCAcquisitionWindow=15  SOCTriggerSource=ePWM1_ADCSOCA  SOCInterruptTrigger=No ADCINT  Ts=-1  dType=uint16  postInterrupt=on  interruptSel=ADCINT1  ADCINTContinuous=on  endma=off  chdma=1  conv1=ADCINA0  conv2=ADCINA0 and ADCINB0  conv1_Type4=ADCIN3  conv2_Type4=ADCIN0 and ADCIN1
      settings: LibrarySourceBlock=c2837xDlib/ADC
  Calibrate_Ir : Subsystem  mask{Offset=(3.3/3)*2047, Gain=1.65/(2047*0.007*20*10)}
  Calibrate_Is : Subsystem  mask{Offset=2047, Gain=1.65/(2047*0.007*20*10)}
  Calibrate_It : Subsystem  mask{Offset=2047, Gain=1.65/(2047*0.007*20*10)}
  Calibrate_Vdc : Subsystem  mask{Offset=(3.3/3)*2048, Gain=(67.0/5.0)*(3/4095.0)}
  Demux : Demux  Outputs=3
  Moving Average Filter1 : Subsystem  mask{N=40}
      mask prompts: N "Order of Filter"
  Position Measurement : Subsystem
  Terminator{,1..3} (4 alike) : Terminator
  w calculation : Subsystem
  Vdc : Outport
  Ir : Outport  Port=2
  Is : Outport  Port=3
  It : Outport  Port=4
  w : Outport  Port=5
  wires:
  ADC2/1 -> Calibrate_It/1(In Raw)
  w calculation/1(w) -> w/1
  Calibrate_Is/1(Out Calibrated) -> Is/1
  Calibrate_It/1(Out Calibrated) -> It/1
  Position Measurement/1(Theta_e) -> w calculation/1(Pos)  "Pos"
  ADC/1 -> Calibrate_Ir/1(In Raw)
  Calibrate_Ir/1(Out Calibrated) -> Ir/1
  ADC1/1 -> Calibrate_Is/1(In Raw)
  Feedback/1 -> Demux/1  "Feedback"
  Demux/1 -> Terminator/1
  Demux/2 -> Terminator1/1
  Demux/3 -> Terminator2/1
  Moving Average Filter1/1(Filtered Out) -> Terminator3/1  "Vdc_Filtered"
  ADC3/1 -> Calibrate_Vdc/1(In Raw)
  Calibrate_Vdc/1(Out Calibrated) -> Moving Average Filter1/1(In Raw), Vdc/1

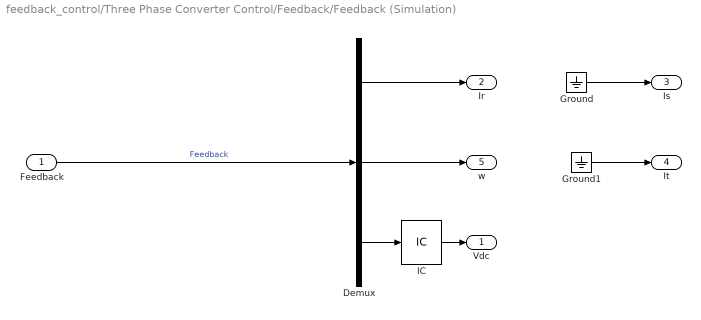
== system feedback_control/Three Phase Converter Control/Feedback/Feedback (Simulation) ==
  Feedback : Inport
  Demux : Demux  Outputs=3
  Ground : Ground
  Ground1 : Ground
  IC : InitialCondition  Value=24
  Vdc : Outport
  Ir : Outport  Port=2
  Is : Outport  Port=3
  It : Outport  Port=4
  w : Outport  Port=5
  wires:
  Feedback/1 -> Demux/1  "Feedback"
  Ground/1 -> Is/1
  Ground1/1 -> It/1
  Demux/1 -> Ir/1
  Demux/3 -> IC/1
  Demux/2 -> w/1
  IC/1 -> Vdc/1

== system feedback_control/Hardware Init/HW_Init/HW_Init (Codegen)/Enable DRV8305 for motor 1 ==
  note: It sets the Current Sense Amplifier to a Gain o 8. The range the current is:
      | ADC Range = +- 2.4125A wrt 0-4095 counts
  6PWM_Mode : Constant  Priority=1000  Commented=on  Value=0x3A16  OutDataTypeStr=uint16  SampleTime=-1
  ADC_Gain_Setting : Constant  Priority=1000  Value=0x503F  OutDataTypeStr=uint16  SampleTime=-1
  Display : Display  Commented=on
      settings: Format=hex (Stored Integer)
  Display1 : Display
      settings: Format=hex (Stored Integer)
  SPI Master Transfer : c280xlib/SPI Controller Transfer  Commented=on  SPISelect=SPI_A  ClockPolarity=Rising_edge  ClockPhase=No_delay  SPIModule=uint32(0)  Mode=Master  BusSpeed=uint32(1000000)  FirstBitToTransfer=Most significant bit (MSB)  ClockMode=0  BlockFunction=Transfer  EnableRegisterAddress=off  RegisterAddress=0  OutputDataType=int8  OutputDataLength=1  DataBits=16  UseCustomSSPin=Provided by the SPI peripheral  ActiveLowSSPin=Active low  Pin=61
  SPI Master Transfer1 : c280xlib/SPI Controller Transfer  SPISelect=SPI_A  ClockPolarity=Rising_edge  ClockPhase=No_delay  SPIModule=uint32(0)  Mode=Master  BusSpeed=uint32(1000000)  FirstBitToTransfer=Most significant bit (MSB)  ClockMode=0  BlockFunction=Transfer  EnableRegisterAddress=off  RegisterAddress=0  OutputDataType=int8  OutputDataLength=1  DataBits=16  UseCustomSSPin=Provided by the SPI peripheral  ActiveLowSSPin=Active low  Pin=61
  wires:
  6PWM_Mode/1 -> SPI Master Transfer/1
  ADC_Gain_Setting/1 -> SPI Master Transfer1/1
  SPI Master Transfer1/1 -> Display1/1
  SPI Master Transfer/1 -> Display/1

== system feedback_control/Three Phase Converter Control/Feedback/ADC Channels/Calibrate_Ir ==
  In Raw : Inport
  Add : Sum  Inputs=+-
  Data Type Conversion : DataTypeConversion  SaturateOnIntegerOverflow=off  RndMeth=Floor
  Gain1 : Gain  Gain=Gain  OutDataTypeStr=single
  Offset : Constant  Value=Offset  OutDataTypeStr=single  SampleTime=-1
  Out Calibrated : Outport
  wires:
  Offset/1 -> Add/2
  Add/1 -> Gain1/1
  In Raw/1 -> Data Type Conversion/1
  Gain1/1 -> Out Calibrated/1
  Data Type Conversion/1 -> Add/1

== system feedback_control/Three Phase Converter Control/Feedback/ADC Channels/Calibrate_Is ==
  In Raw : Inport
  Add : Sum  Inputs=+-
  Gain1 : Gain  Gain=Gain  OutDataTypeStr=single
  Offset : Constant  Value=Offset  OutDataTypeStr=single  SampleTime=-1
  Out Calibrated : Outport
  wires:
  Gain1/1 -> Out Calibrated/1
  In Raw/1 -> Add/1
  Add/1 -> Gain1/1
  Offset/1 -> Add/2

== system feedback_control/Three Phase Converter Control/Feedback/ADC Channels/Calibrate_It ==
  In Raw : Inport
  Add : Sum  Inputs=+-
  Gain1 : Gain  Gain=Gain  OutDataTypeStr=single
  Offset : Constant  Value=Offset  OutDataTypeStr=single  SampleTime=-1
  Out Calibrated : Outport
  wires:
  Offset/1 -> Add/2
  Add/1 -> Gain1/1
  In Raw/1 -> Add/1
  Gain1/1 -> Out Calibrated/1

== system feedback_control/Three Phase Converter Control/Feedback/ADC Channels/Calibrate_Vdc ==
  In Raw : Inport
  Add : Sum  Inputs=+-
  Data Type Conversion : DataTypeConversion  SaturateOnIntegerOverflow=off  RndMeth=Floor
  Gain1 : Gain  Gain=Gain  OutDataTypeStr=single
  Offset : Constant  Value=Offset  OutDataTypeStr=single  SampleTime=-1
  Out Calibrated : Outport
  wires:
  Gain1/1 -> Out Calibrated/1
  In Raw/1 -> Data Type Conversion/1
  Add/1 -> Gain1/1
  Offset/1 -> Add/2
  Data Type Conversion/1 -> Add/1

== system feedback_control/Three Phase Converter Control/Feedback/ADC Channels/Moving Average Filter1 ==
  note: This is an Average Moving Filter, which order can be changed in real time. The only purpose of this fiter is in order to:
      |
      | 1.- Increase resolution of the measure.
      | 2.- Improve the readibility of the magnitude, which change continuosly at a high freqüency, and thanks to this filter, the reading keeps more constant.
  In Raw : Inport
  Matrix Concatenate : Concatenate  NumInputs=1  Mode=Multidimensional array  ConcatenateDimension=N
  Sum of Elements : Sum  Inputs=+
  Unit Delay : UnitDelay  SampleTime=-1  HasFrameUpgradeWarning=on
  Filtered Out : Outport
  wires:
  Matrix Concatenate/1 -> Sum of Elements/1
  In Raw/1 -> Unit Delay/1
  Unit Delay/1 -> Matrix Concatenate/1
  Sum of Elements/1 -> Filtered Out/1

== system feedback_control/Three Phase Converter Control/Feedback/ADC Channels/Position Measurement ==
  "Calculate Position from QEP count " : Subsystem
  eQEP : c280xlib/eQEP  useModule=eQEP1  pcInputmode=Quadrature-count  externalClockrate=2x resolution: Count the rising/falling edge  swapPolarityselection=Clockwise  qdfOutputport=off  qapPolarityselection=on  qbpPolarityselection=on  qipPolarityselection=on  qspPolarityselection=off  igatePolarityselection=off  sampleTime=-1  pcOutputport=on  pcMaximumvalue=2^16-1  indexInitializationcheck=off  indexInitializationevent=Falling edge  strobeInitializationcheck=off  strobeInitializationevent=Rising edge  softwareInitializationcheck=off  softwareInitializationsource=Set to init value at start up  softwareInitializationmode=on  pcInitialvalue=0  pcResetmode=Reset on the first index event  ieloutputport=on  indexEventlatch=Falling edge  seloutputport=off  strobeEventlatch=Rising edge  pcefOutputport=off  enableEqepcapture=off  qctmrOutputport=off  qcprdOutputport=off  captureTimerprescaler=128  upEventprescaler=128  overflowErrorflag=off  directionErrorflag=off  captureTimerposition=On position counter read  unitTimerperiod=100000000  captureTimerlatch=off  capturePeriodlatch=off  positionCounterlatch=off  soenPolarityselection=off  spselPolarityselection=Index pin is used for sync output  compareValuesource=Specify via dialog  shadowMode=Load on QPOSCNT=0  compareValue=4294967295  syncOutputwidth=1  polaritySyncoutput=Active high  watchdogEnable=off  watchdogTimer=65535  outport1Datatype=auto  outport2Datatype=auto  outport3Datatype=auto  outport4Datatype=auto  outport5Datatype=auto  outport6Datatype=auto  outport7Datatype=auto  outport8Datatype=auto  outport9Datatype=auto  outport10Datatype=auto  outport11Datatype=auto  outport12Datatype=auto  eqepinterrupt_pce=off  eqepinterrupt_qpe=off  eqepinterrupt_qdc=off  eqepinterrupt_wto=off  eqepinterrupt_pcu=off  eqepinterrupt_pco=off  eqepinterrupt_pcr=off  eqepinterrupt_pcm=off  eqepinterrupt_sel=off  eqepinterrupt_iel=off  eqepinterrupt_uto=off  pheOutputport=off  watchdogOutputport=off  outport13Datatype=auto  outport14Datatype=auto
  Theta_e : Outport
  wires:
  eQEP/1 -> "Calculate Position from QEP count "/1(Count)
  eQEP/2 -> "Calculate Position from QEP count "/2(Index)
  "Calculate Position from QEP count "/1(Theta_e) -> Theta_e/1

== system feedback_control/Three Phase Converter Control/Feedback/ADC Channels/w calculation ==
  Pos : Inport
  Add : Sum  Inputs=+-
  Gain : Gain  Gain=1/T_sample_control
  Unit Delay : UnitDelay  SampleTime=-1  HasFrameUpgradeWarning=on
  w : Outport
  wires:
  Pos/1 -> Unit Delay/1, Add/1
  Unit Delay/1 -> Add/2
  Add/1 -> Gain/1
  Gain/1 -> w/1

== system feedback_control/Three Phase Converter Control/Feedback/ADC Channels/Position Measurement/Calculate Position from QEP count  ==
  Count : Inport
  Index : Inport  Port=2
  eQEP_Decoder : Subsystem
  Theta_e : Outport  InitialOutput=0  VectorParamsAs1DForOutWhenUnconnected=off
  wires:
  Index/1 -> eQEP_Decoder/2(Index)
  Count/1 -> eQEP_Decoder/1(Count)
  eQEP_Decoder/1(Theta_e) -> Theta_e/1

== system feedback_control/Three Phase Converter Control/Feedback/ADC Channels/Position Measurement/Calculate Position from QEP count /eQEP_Decoder ==
  Count : Inport
  Index : Inport  Port=2
  Mechanical to Electrical Position : mcbpositiondecoderlib/Mechanical to Electrical Position  PolePairsInputType=Specify via dialog  NrPP=4  selectedRange=Per unit  MechOfstInputType=Specify via dialog  mechOffsetIn=0  maxAngleIn=1  InputDataType=single  VariantSelect=floating-point
  Quadrature Decoder : mcbpositiondecoderlib/Quadrature Decoder  EncoderSlitsPerRevolution=4000  EncoderCountsPerSlit=4  CounterSize=16 bits  ExternalIndexCount=on  PositionUnit=Per unit  PositionDataType=single  ParameterInputType=off  CountsPerRevInverseDataType=single
  Theta_e : Outport  VectorParamsAs1DForOutWhenUnconnected=off
  wires:
  Count/1 -> Quadrature Decoder/1
  Index/1 -> Quadrature Decoder/2
  Mechanical to Electrical Position/1 -> Theta_e/1
  Quadrature Decoder/1 -> Mechanical to Electrical Position/1
